simulink model "MMADC"  (R2021a)
settings: Solver=VariableStepAuto  StartTime=0.0  StopTime=1  RelTol=1e-3
values from neighbouring files (symbols this model uses):
  Cf = minimum_cap    [MMADC_main.m]
  clk_freq = 2.1*(nb_MAC+1)/nb_MAC*input_BW    (= 1684.375)    [MMADC_main.m]
  clk_period = 1/clk_freq    (= 0.000593692022263)    [MMADC_main.m]
  comparator_high_offset = 0.2*10e-4    (= 0.0002)    [MMADC_main.m]
  comparator_low_offset = -.1*10e-4    (= -0.0001)    [MMADC_main.m]
  comparator_noise_on = noise_on    (= 1)    [MMADC_main.m]
  comparator_noise_rms = 1*k*T* 2/3 / minimum_cap    [MMADC_main.m]
  comparator_offset_on = noise_on    (= 1)    [MMADC_main.m]
  k = 1.38064852e-23    [MMADC_main.m]
  LNA_bandwidth = 2.5*input_BW    (= 2000)    [MMADC_main.m]
  LNA_gain = 10^(36/20)*12*1.5849    (= 1200.00515432)    [MMADC_main.m]
  LNA_input_referred_noise = sqrt(pi/2*LNA_bandwidth*(194*10^-9)^2)    [MMADC_main.m]
  LNA_noise_on = noise_on    (= 1)    [MMADC_main.m]
  MM_incomplete_transfer_coeff = C1/(C1+C2)    [MMADC_main.m]
  MM_leakage_per_clk_cycle = 1    [MMADC_main.m]
  MM_sampling_noise = noise_on*((k*T * C1/(C1+C2)^2) + (k*T*(C1*C2/(C1+C2))/C2^2))    [MMADC_main.m]
  nb_MAC = 384    [MMADC_main.m]
  number_of_bits = 6    [MMADC_main.m]
  sample_time_jitter = 16e-12    (= 1.6e-11)    [MMADC_main.m]
  sampling_gain = Cs/Cf    [MMADC_main.m]
  sampling_jitter_on = noise_on    (= 1)    [MMADC_main.m]
  sensing_matrix = sensing_matrix_large(j:j+min(19,i-1),:)    [MMADC_main.m]
  sim_number = 0    [MMADC_main.m]
  switch_noise_on = noise_on    (= 1)    [MMADC_main.m]
  switching_noise = k*T/Cf    [MMADC_main.m]
  T = 293    [MMADC_main.m]
  Vref = 2    [MMADC_main.m]
  ZOH_delta = 0*Vref/(2^number_of_bits)    (= 0)    [MMADC_main.m]
libraries: simulink x100, simulink_extras x41, dspsigops x21, dspsrcs4 x21, spsFirstOrderFilterLib x1, dspswit3 x1
(part 9 of 10)

== system MMADC/Sensing Channel 2/SAR/ZOH+comparator/Old parallel ZOH comparator/Signal>DAC? ==
  y(t) : Inport
  DAC_in : Inport  Port=2
  Trigger : TriggerPort  VariantControl=Variant
  Add : Sum
  Add1 : Sum
  Compare To Zero : simulink/Logic and Bit Operations/Compare To Zero  relop=>  OutDataTypeStr=boolean
  Constant : Constant  Value=comparator_high_offset
  Constant1 : Constant  Value=comparator_low_offset
  Constant2 : Constant  Value=0
  Constant3 : Constant  Value=comparator_offset_on
  Constant4 : Constant  Value=0
  Constant5 : Constant  Value=comparator_noise_on
  Multiply : Gain  Gain=comparator_noise_rms
  Random Number : RandomNumber
  Subtract : Sum  Inputs=+-
  Switch : Switch  Criteria=u2 > Threshold
  Switch1 : Switch  Criteria=u2 > Threshold
  Switch2 : Switch  Criteria=u2 > Threshold
  Unit Delay : UnitDelay  SampleTime=-1  HasFrameUpgradeWarning=on
  Comparator_out : Outport
  wires:
  Switch/1 -> Switch1/1
  Subtract/1 -> Add/1
  Constant/1 -> Switch/1
  Constant2/1 -> Switch1/3
  Add/1 -> Compare To Zero/1
  Switch1/1 -> Add/2
  Compare To Zero/1 -> Unit Delay/1, Comparator_out/1
  Constant3/1 -> Switch1/2
  Unit Delay/1 -> Switch/2
  Constant1/1 -> Switch/3
  DAC_in/1 -> Subtract/2
  Add1/1 -> Subtract/1
  y(t)/1 -> Add1/2
  Random Number/1 -> Multiply/1
  Switch2/1 -> Add1/1
  Multiply/1 -> Switch2/1
  Constant4/1 -> Switch2/3
  Constant5/1 -> Switch2/2

== system MMADC/Sensing Channel 20/SAR/ZOH+comparator/Old parallel ZOH comparator/ DAC-signal < delta? ==
  y(t) : Inport
  DAC_in : Inport  Port=2
  Trigger : TriggerPort  VariantControl=Variant
  Add : Sum
  Add1 : Sum
  Compare To Zero : simulink/Logic and Bit Operations/Compare To Zero  relop=>  OutDataTypeStr=boolean
  Constant : Constant  Value=comparator_high_offset
  Constant1 : Constant  Value=comparator_low_offset
  Constant2 : Constant  Value=0
  Constant3 : Constant  Value=comparator_offset_on
  Constant4 : Constant  Value=0
  Constant5 : Constant  Value=comparator_noise_on
  Multiply : Gain  Gain=comparator_noise_rms
  Random Number : RandomNumber
  Subtract : Sum  Inputs=+-
  Switch : Switch  Criteria=u2 > Threshold
  Switch1 : Switch  Criteria=u2 > Threshold
  Switch2 : Switch  Criteria=u2 > Threshold
  Unit Delay : UnitDelay  SampleTime=-1  HasFrameUpgradeWarning=on
  Comparator_out : Outport
  wires:
  Switch/1 -> Switch1/1
  Subtract/1 -> Add/1
  Constant/1 -> Switch/1
  Constant2/1 -> Switch1/3
  Add/1 -> Compare To Zero/1
  Switch1/1 -> Add/2
  Compare To Zero/1 -> Unit Delay/1, Comparator_out/1
  Constant3/1 -> Switch1/2
  Unit Delay/1 -> Switch/2
  Constant1/1 -> Switch/3
  DAC_in/1 -> Subtract/2
  Add1/1 -> Subtract/1
  y(t)/1 -> Add1/2
  Random Number/1 -> Multiply/1
  Switch2/1 -> Add1/1
  Multiply/1 -> Switch2/1
  Constant4/1 -> Switch2/3
  Constant5/1 -> Switch2/2

== system MMADC/Sensing Channel 20/SAR/ZOH+comparator/Old parallel ZOH comparator/Count ZOH's ==
  In1 : Inport
  Trigger : TriggerPort  VariantControl=Variant  PortDimensions=1
  Add : Sum  AccumDataTypeStr=double  OutDataTypeStr=double
  Unit Delay : UnitDelay  SampleTime=-1  HasFrameUpgradeWarning=on
  Out1 : Outport
  wires:
  In1/1 -> Add/1
  Add/1 -> Unit Delay/1, Out1/1
  Unit Delay/1 -> Add/2

== system MMADC/Sensing Channel 20/SAR/ZOH+comparator/Old parallel ZOH comparator/Signal-DAC < delta? ==
  y(t) : Inport
  DAC_in : Inport  Port=2
  Trigger : TriggerPort  VariantControl=Variant
  Add : Sum
  Add1 : Sum
  Compare To Zero : simulink/Logic and Bit Operations/Compare To Zero  relop=>  OutDataTypeStr=boolean
  Constant : Constant  Value=comparator_high_offset
  Constant1 : Constant  Value=comparator_low_offset
  Constant2 : Constant  Value=0
  Constant3 : Constant  Value=comparator_offset_on
  Constant4 : Constant  Value=0
  Constant5 : Constant  Value=comparator_noise_on
  Multiply : Gain  Gain=comparator_noise_rms
  Random Number : RandomNumber
  Subtract : Sum  Inputs=+-
  Switch : Switch  Criteria=u2 > Threshold
  Switch1 : Switch  Criteria=u2 > Threshold
  Switch2 : Switch  Criteria=u2 > Threshold
  Unit Delay : UnitDelay  SampleTime=-1  HasFrameUpgradeWarning=on
  Comparator_out : Outport
  wires:
  Switch/1 -> Switch1/1
  Subtract/1 -> Add/1
  Constant/1 -> Switch/1
  Constant2/1 -> Switch1/3
  Add/1 -> Compare To Zero/1
  Switch1/1 -> Add/2
  Compare To Zero/1 -> Unit Delay/1, Comparator_out/1
  Constant3/1 -> Switch1/2
  Unit Delay/1 -> Switch/2
  Constant1/1 -> Switch/3
  DAC_in/1 -> Subtract/2
  Add1/1 -> Subtract/1
  y(t)/1 -> Add1/2
  Random Number/1 -> Multiply/1
  Switch2/1 -> Add1/1
  Multiply/1 -> Switch2/1
  Constant4/1 -> Switch2/3
  Constant5/1 -> Switch2/2

== system MMADC/Sensing Channel 20/SAR/ZOH+comparator/Old parallel ZOH comparator/Signal>DAC? ==
  y(t) : Inport
  DAC_in : Inport  Port=2
  Trigger : TriggerPort  VariantControl=Variant
  Add : Sum
  Add1 : Sum
  Compare To Zero : simulink/Logic and Bit Operations/Compare To Zero  relop=>  OutDataTypeStr=boolean
  Constant : Constant  Value=comparator_high_offset
  Constant1 : Constant  Value=comparator_low_offset
  Constant2 : Constant  Value=0
  Constant3 : Constant  Value=comparator_offset_on
  Constant4 : Constant  Value=0
  Constant5 : Constant  Value=comparator_noise_on
  Multiply : Gain  Gain=comparator_noise_rms
  Random Number : RandomNumber
  Subtract : Sum  Inputs=+-
  Switch : Switch  Criteria=u2 > Threshold
  Switch1 : Switch  Criteria=u2 > Threshold
  Switch2 : Switch  Criteria=u2 > Threshold
  Unit Delay : UnitDelay  SampleTime=-1  HasFrameUpgradeWarning=on
  Comparator_out : Outport
  wires:
  Switch/1 -> Switch1/1
  Subtract/1 -> Add/1
  Constant/1 -> Switch/1
  Constant2/1 -> Switch1/3
  Add/1 -> Compare To Zero/1
  Switch1/1 -> Add/2
  Compare To Zero/1 -> Unit Delay/1, Comparator_out/1
  Constant3/1 -> Switch1/2
  Unit Delay/1 -> Switch/2
  Constant1/1 -> Switch/3
  DAC_in/1 -> Subtract/2
  Add1/1 -> Subtract/1
  y(t)/1 -> Add1/2
  Random Number/1 -> Multiply/1
  Switch2/1 -> Add1/1
  Multiply/1 -> Switch2/1
  Constant4/1 -> Switch2/3
  Constant5/1 -> Switch2/2

== system MMADC/Sensing Channel 3/SAR/ZOH+comparator/Old parallel ZOH comparator/ DAC-signal < delta? ==
  y(t) : Inport
  DAC_in : Inport  Port=2
  Trigger : TriggerPort  VariantControl=Variant
  Add : Sum
  Add1 : Sum
  Compare To Zero : simulink/Logic and Bit Operations/Compare To Zero  relop=>  OutDataTypeStr=boolean
  Constant : Constant  Value=comparator_high_offset
  Constant1 : Constant  Value=comparator_low_offset
  Constant2 : Constant  Value=0
  Constant3 : Constant  Value=comparator_offset_on
  Constant4 : Constant  Value=0
  Constant5 : Constant  Value=comparator_noise_on
  Multiply : Gain  Gain=comparator_noise_rms
  Random Number : RandomNumber
  Subtract : Sum  Inputs=+-
  Switch : Switch  Criteria=u2 > Threshold
  Switch1 : Switch  Criteria=u2 > Threshold
  Switch2 : Switch  Criteria=u2 > Threshold
  Unit Delay : UnitDelay  SampleTime=-1  HasFrameUpgradeWarning=on
  Comparator_out : Outport
  wires:
  Switch/1 -> Switch1/1
  Subtract/1 -> Add/1
  Constant/1 -> Switch/1
  Constant2/1 -> Switch1/3
  Add/1 -> Compare To Zero/1
  Switch1/1 -> Add/2
  Compare To Zero/1 -> Unit Delay/1, Comparator_out/1
  Constant3/1 -> Switch1/2
  Unit Delay/1 -> Switch/2
  Constant1/1 -> Switch/3
  DAC_in/1 -> Subtract/2
  Add1/1 -> Subtract/1
  y(t)/1 -> Add1/2
  Random Number/1 -> Multiply/1
  Switch2/1 -> Add1/1
  Multiply/1 -> Switch2/1
  Constant4/1 -> Switch2/3
  Constant5/1 -> Switch2/2

== system MMADC/Sensing Channel 3/SAR/ZOH+comparator/Old parallel ZOH comparator/Count ZOH's ==
  In1 : Inport
  Trigger : TriggerPort  VariantControl=Variant  PortDimensions=1
  Add : Sum  AccumDataTypeStr=double  OutDataTypeStr=double
  Unit Delay : UnitDelay  SampleTime=-1  HasFrameUpgradeWarning=on
  Out1 : Outport
  wires:
  In1/1 -> Add/1
  Add/1 -> Unit Delay/1, Out1/1
  Unit Delay/1 -> Add/2

== system MMADC/Sensing Channel 3/SAR/ZOH+comparator/Old parallel ZOH comparator/Signal-DAC < delta? ==
  y(t) : Inport
  DAC_in : Inport  Port=2
  Trigger : TriggerPort  VariantControl=Variant
  Add : Sum
  Add1 : Sum
  Compare To Zero : simulink/Logic and Bit Operations/Compare To Zero  relop=>  OutDataTypeStr=boolean
  Constant : Constant  Value=comparator_high_offset
  Constant1 : Constant  Value=comparator_low_offset
  Constant2 : Constant  Value=0
  Constant3 : Constant  Value=comparator_offset_on
  Constant4 : Constant  Value=0
  Constant5 : Constant  Value=comparator_noise_on
  Multiply : Gain  Gain=comparator_noise_rms
  Random Number : RandomNumber
  Subtract : Sum  Inputs=+-
  Switch : Switch  Criteria=u2 > Threshold
  Switch1 : Switch  Criteria=u2 > Threshold
  Switch2 : Switch  Criteria=u2 > Threshold
  Unit Delay : UnitDelay  SampleTime=-1  HasFrameUpgradeWarning=on
  Comparator_out : Outport
  wires:
  Switch/1 -> Switch1/1
  Subtract/1 -> Add/1
  Constant/1 -> Switch/1
  Constant2/1 -> Switch1/3
  Add/1 -> Compare To Zero/1
  Switch1/1 -> Add/2
  Compare To Zero/1 -> Unit Delay/1, Comparator_out/1
  Constant3/1 -> Switch1/2
  Unit Delay/1 -> Switch/2
  Constant1/1 -> Switch/3
  DAC_in/1 -> Subtract/2
  Add1/1 -> Subtract/1
  y(t)/1 -> Add1/2
  Random Number/1 -> Multiply/1
  Switch2/1 -> Add1/1
  Multiply/1 -> Switch2/1
  Constant4/1 -> Switch2/3
  Constant5/1 -> Switch2/2

== system MMADC/Sensing Channel 3/SAR/ZOH+comparator/Old parallel ZOH comparator/Signal>DAC? ==
  y(t) : Inport
  DAC_in : Inport  Port=2
  Trigger : TriggerPort  VariantControl=Variant
  Add : Sum
  Add1 : Sum
  Compare To Zero : simulink/Logic and Bit Operations/Compare To Zero  relop=>  OutDataTypeStr=boolean
  Constant : Constant  Value=comparator_high_offset
  Constant1 : Constant  Value=comparator_low_offset
  Constant2 : Constant  Value=0
  Constant3 : Constant  Value=comparator_offset_on
  Constant4 : Constant  Value=0
  Constant5 : Constant  Value=comparator_noise_on
  Multiply : Gain  Gain=comparator_noise_rms
  Random Number : RandomNumber
  Subtract : Sum  Inputs=+-
  Switch : Switch  Criteria=u2 > Threshold
  Switch1 : Switch  Criteria=u2 > Threshold
  Switch2 : Switch  Criteria=u2 > Threshold
  Unit Delay : UnitDelay  SampleTime=-1  HasFrameUpgradeWarning=on
  Comparator_out : Outport
  wires:
  Switch/1 -> Switch1/1
  Subtract/1 -> Add/1
  Constant/1 -> Switch/1
  Constant2/1 -> Switch1/3
  Add/1 -> Compare To Zero/1
  Switch1/1 -> Add/2
  Compare To Zero/1 -> Unit Delay/1, Comparator_out/1
  Constant3/1 -> Switch1/2
  Unit Delay/1 -> Switch/2
  Constant1/1 -> Switch/3
  DAC_in/1 -> Subtract/2
  Add1/1 -> Subtract/1
  y(t)/1 -> Add1/2
  Random Number/1 -> Multiply/1
  Switch2/1 -> Add1/1
  Multiply/1 -> Switch2/1
  Constant4/1 -> Switch2/3
  Constant5/1 -> Switch2/2

== system MMADC/Sensing Channel 4/SAR/ZOH+comparator/Old parallel ZOH comparator/ DAC-signal < delta? ==
  y(t) : Inport
  DAC_in : Inport  Port=2
  Trigger : TriggerPort  VariantControl=Variant
  Add : Sum
  Add1 : Sum
  Compare To Zero : simulink/Logic and Bit Operations/Compare To Zero  relop=>  OutDataTypeStr=boolean
  Constant : Constant  Value=comparator_high_offset
  Constant1 : Constant  Value=comparator_low_offset
  Constant2 : Constant  Value=0
  Constant3 : Constant  Value=comparator_offset_on
  Constant4 : Constant  Value=0
  Constant5 : Constant  Value=comparator_noise_on
  Multiply : Gain  Gain=comparator_noise_rms
  Random Number : RandomNumber
  Subtract : Sum  Inputs=+-
  Switch : Switch  Criteria=u2 > Threshold
  Switch1 : Switch  Criteria=u2 > Threshold
  Switch2 : Switch  Criteria=u2 > Threshold
  Unit Delay : UnitDelay  SampleTime=-1  HasFrameUpgradeWarning=on
  Comparator_out : Outport
  wires:
  Switch/1 -> Switch1/1
  Subtract/1 -> Add/1
  Constant/1 -> Switch/1
  Constant2/1 -> Switch1/3
  Add/1 -> Compare To Zero/1
  Switch1/1 -> Add/2
  Compare To Zero/1 -> Unit Delay/1, Comparator_out/1
  Constant3/1 -> Switch1/2
  Unit Delay/1 -> Switch/2
  Constant1/1 -> Switch/3
  DAC_in/1 -> Subtract/2
  Add1/1 -> Subtract/1
  y(t)/1 -> Add1/2
  Random Number/1 -> Multiply/1
  Switch2/1 -> Add1/1
  Multiply/1 -> Switch2/1
  Constant4/1 -> Switch2/3
  Constant5/1 -> Switch2/2

== system MMADC/Sensing Channel 4/SAR/ZOH+comparator/Old parallel ZOH comparator/Count ZOH's ==
  In1 : Inport
  Trigger : TriggerPort  VariantControl=Variant  PortDimensions=1
  Add : Sum  AccumDataTypeStr=double  OutDataTypeStr=double
  Unit Delay : UnitDelay  SampleTime=-1  HasFrameUpgradeWarning=on
  Out1 : Outport
  wires:
  In1/1 -> Add/1
  Add/1 -> Unit Delay/1, Out1/1
  Unit Delay/1 -> Add/2

== system MMADC/Sensing Channel 4/SAR/ZOH+comparator/Old parallel ZOH comparator/Signal-DAC < delta? ==
  y(t) : Inport
  DAC_in : Inport  Port=2
  Trigger : TriggerPort  VariantControl=Variant
  Add : Sum
  Add1 : Sum
  Compare To Zero : simulink/Logic and Bit Operations/Compare To Zero  relop=>  OutDataTypeStr=boolean
  Constant : Constant  Value=comparator_high_offset
  Constant1 : Constant  Value=comparator_low_offset
  Constant2 : Constant  Value=0
  Constant3 : Constant  Value=comparator_offset_on
  Constant4 : Constant  Value=0
  Constant5 : Constant  Value=comparator_noise_on
  Multiply : Gain  Gain=comparator_noise_rms
  Random Number : RandomNumber
  Subtract : Sum  Inputs=+-
  Switch : Switch  Criteria=u2 > Threshold
  Switch1 : Switch  Criteria=u2 > Threshold
  Switch2 : Switch  Criteria=u2 > Threshold
  Unit Delay : UnitDelay  SampleTime=-1  HasFrameUpgradeWarning=on
  Comparator_out : Outport
  wires:
  Switch/1 -> Switch1/1
  Subtract/1 -> Add/1
  Constant/1 -> Switch/1
  Constant2/1 -> Switch1/3
  Add/1 -> Compare To Zero/1
  Switch1/1 -> Add/2
  Compare To Zero/1 -> Unit Delay/1, Comparator_out/1
  Constant3/1 -> Switch1/2
  Unit Delay/1 -> Switch/2
  Constant1/1 -> Switch/3
  DAC_in/1 -> Subtract/2
  Add1/1 -> Subtract/1
  y(t)/1 -> Add1/2
  Random Number/1 -> Multiply/1
  Switch2/1 -> Add1/1
  Multiply/1 -> Switch2/1
  Constant4/1 -> Switch2/3
  Constant5/1 -> Switch2/2

== system MMADC/Sensing Channel 4/SAR/ZOH+comparator/Old parallel ZOH comparator/Signal>DAC? ==
  y(t) : Inport
  DAC_in : Inport  Port=2
  Trigger : TriggerPort  VariantControl=Variant
  Add : Sum
  Add1 : Sum
  Compare To Zero : simulink/Logic and Bit Operations/Compare To Zero  relop=>  OutDataTypeStr=boolean
  Constant : Constant  Value=comparator_high_offset
  Constant1 : Constant  Value=comparator_low_offset
  Constant2 : Constant  Value=0
  Constant3 : Constant  Value=comparator_offset_on
  Constant4 : Constant  Value=0
  Constant5 : Constant  Value=comparator_noise_on
  Multiply : Gain  Gain=comparator_noise_rms
  Random Number : RandomNumber
  Subtract : Sum  Inputs=+-
  Switch : Switch  Criteria=u2 > Threshold
  Switch1 : Switch  Criteria=u2 > Threshold
  Switch2 : Switch  Criteria=u2 > Threshold
  Unit Delay : UnitDelay  SampleTime=-1  HasFrameUpgradeWarning=on
  Comparator_out : Outport
  wires:
  Switch/1 -> Switch1/1
  Subtract/1 -> Add/1
  Constant/1 -> Switch/1
  Constant2/1 -> Switch1/3
  Add/1 -> Compare To Zero/1
  Switch1/1 -> Add/2
  Compare To Zero/1 -> Unit Delay/1, Comparator_out/1
  Constant3/1 -> Switch1/2
  Unit Delay/1 -> Switch/2
  Constant1/1 -> Switch/3
  DAC_in/1 -> Subtract/2
  Add1/1 -> Subtract/1
  y(t)/1 -> Add1/2
  Random Number/1 -> Multiply/1
  Switch2/1 -> Add1/1
  Multiply/1 -> Switch2/1
  Constant4/1 -> Switch2/3
  Constant5/1 -> Switch2/2

== system MMADC/Sensing Channel 5/SAR/ZOH+comparator/Old parallel ZOH comparator/ DAC-signal < delta? ==
  y(t) : Inport
  DAC_in : Inport  Port=2
  Trigger : TriggerPort  VariantControl=Variant
  Add : Sum
  Add1 : Sum
  Compare To Zero : simulink/Logic and Bit Operations/Compare To Zero  relop=>  OutDataTypeStr=boolean
  Constant : Constant  Value=comparator_high_offset
  Constant1 : Constant  Value=comparator_low_offset
  Constant2 : Constant  Value=0
  Constant3 : Constant  Value=comparator_offset_on
  Constant4 : Constant  Value=0
  Constant5 : Constant  Value=comparator_noise_on
  Multiply : Gain  Gain=comparator_noise_rms
  Random Number : RandomNumber
  Subtract : Sum  Inputs=+-
  Switch : Switch  Criteria=u2 > Threshold
  Switch1 : Switch  Criteria=u2 > Threshold
  Switch2 : Switch  Criteria=u2 > Threshold
  Unit Delay : UnitDelay  SampleTime=-1  HasFrameUpgradeWarning=on
  Comparator_out : Outport
  wires:
  Switch/1 -> Switch1/1
  Subtract/1 -> Add/1
  Constant/1 -> Switch/1
  Constant2/1 -> Switch1/3
  Add/1 -> Compare To Zero/1
  Switch1/1 -> Add/2
  Compare To Zero/1 -> Unit Delay/1, Comparator_out/1
  Constant3/1 -> Switch1/2
  Unit Delay/1 -> Switch/2
  Constant1/1 -> Switch/3
  DAC_in/1 -> Subtract/2
  Add1/1 -> Subtract/1
  y(t)/1 -> Add1/2
  Random Number/1 -> Multiply/1
  Switch2/1 -> Add1/1
  Multiply/1 -> Switch2/1
  Constant4/1 -> Switch2/3
  Constant5/1 -> Switch2/2

== system MMADC/Sensing Channel 5/SAR/ZOH+comparator/Old parallel ZOH comparator/Count ZOH's ==
  In1 : Inport
  Trigger : TriggerPort  VariantControl=Variant  PortDimensions=1
  Add : Sum  AccumDataTypeStr=double  OutDataTypeStr=double
  Unit Delay : UnitDelay  SampleTime=-1  HasFrameUpgradeWarning=on
  Out1 : Outport
  wires:
  In1/1 -> Add/1
  Add/1 -> Unit Delay/1, Out1/1
  Unit Delay/1 -> Add/2

== system MMADC/Sensing Channel 5/SAR/ZOH+comparator/Old parallel ZOH comparator/Signal-DAC < delta? ==
  y(t) : Inport
  DAC_in : Inport  Port=2
  Trigger : TriggerPort  VariantControl=Variant
  Add : Sum
  Add1 : Sum
  Compare To Zero : simulink/Logic and Bit Operations/Compare To Zero  relop=>  OutDataTypeStr=boolean
  Constant : Constant  Value=comparator_high_offset
  Constant1 : Constant  Value=comparator_low_offset
  Constant2 : Constant  Value=0
  Constant3 : Constant  Value=comparator_offset_on
  Constant4 : Constant  Value=0
  Constant5 : Constant  Value=comparator_noise_on
  Multiply : Gain  Gain=comparator_noise_rms
  Random Number : RandomNumber
  Subtract : Sum  Inputs=+-
  Switch : Switch  Criteria=u2 > Threshold
  Switch1 : Switch  Criteria=u2 > Threshold
  Switch2 : Switch  Criteria=u2 > Threshold
  Unit Delay : UnitDelay  SampleTime=-1  HasFrameUpgradeWarning=on
  Comparator_out : Outport
  wires:
  Switch/1 -> Switch1/1
  Subtract/1 -> Add/1
  Constant/1 -> Switch/1
  Constant2/1 -> Switch1/3
  Add/1 -> Compare To Zero/1
  Switch1/1 -> Add/2
  Compare To Zero/1 -> Unit Delay/1, Comparator_out/1
  Constant3/1 -> Switch1/2
  Unit Delay/1 -> Switch/2
  Constant1/1 -> Switch/3
  DAC_in/1 -> Subtract/2
  Add1/1 -> Subtract/1
  y(t)/1 -> Add1/2
  Random Number/1 -> Multiply/1
  Switch2/1 -> Add1/1
  Multiply/1 -> Switch2/1
  Constant4/1 -> Switch2/3
  Constant5/1 -> Switch2/2

== system MMADC/Sensing Channel 5/SAR/ZOH+comparator/Old parallel ZOH comparator/Signal>DAC? ==
  y(t) : Inport
  DAC_in : Inport  Port=2
  Trigger : TriggerPort  VariantControl=Variant
  Add : Sum
  Add1 : Sum
  Compare To Zero : simulink/Logic and Bit Operations/Compare To Zero  relop=>  OutDataTypeStr=boolean
  Constant : Constant  Value=comparator_high_offset
  Constant1 : Constant  Value=comparator_low_offset
  Constant2 : Constant  Value=0
  Constant3 : Constant  Value=comparator_offset_on
  Constant4 : Constant  Value=0
  Constant5 : Constant  Value=comparator_noise_on
  Multiply : Gain  Gain=comparator_noise_rms
  Random Number : RandomNumber
  Subtract : Sum  Inputs=+-
  Switch : Switch  Criteria=u2 > Threshold
  Switch1 : Switch  Criteria=u2 > Threshold
  Switch2 : Switch  Criteria=u2 > Threshold
  Unit Delay : UnitDelay  SampleTime=-1  HasFrameUpgradeWarning=on
  Comparator_out : Outport
  wires:
  Switch/1 -> Switch1/1
  Subtract/1 -> Add/1
  Constant/1 -> Switch/1
  Constant2/1 -> Switch1/3
  Add/1 -> Compare To Zero/1
  Switch1/1 -> Add/2
  Compare To Zero/1 -> Unit Delay/1, Comparator_out/1
  Constant3/1 -> Switch1/2
  Unit Delay/1 -> Switch/2
  Constant1/1 -> Switch/3
  DAC_in/1 -> Subtract/2
  Add1/1 -> Subtract/1
  y(t)/1 -> Add1/2
  Random Number/1 -> Multiply/1
  Switch2/1 -> Add1/1
  Multiply/1 -> Switch2/1
  Constant4/1 -> Switch2/3
  Constant5/1 -> Switch2/2

== system MMADC/Sensing Channel 6/SAR/ZOH+comparator/Old parallel ZOH comparator/ DAC-signal < delta? ==
  y(t) : Inport
  DAC_in : Inport  Port=2
  Trigger : TriggerPort  VariantControl=Variant
  Add : Sum
  Add1 : Sum
  Compare To Zero : simulink/Logic and Bit Operations/Compare To Zero  relop=>  OutDataTypeStr=boolean
  Constant : Constant  Value=comparator_high_offset
  Constant1 : Constant  Value=comparator_low_offset
  Constant2 : Constant  Value=0
  Constant3 : Constant  Value=comparator_offset_on
  Constant4 : Constant  Value=0
  Constant5 : Constant  Value=comparator_noise_on
  Multiply : Gain  Gain=comparator_noise_rms
  Random Number : RandomNumber
  Subtract : Sum  Inputs=+-
  Switch : Switch  Criteria=u2 > Threshold
  Switch1 : Switch  Criteria=u2 > Threshold
  Switch2 : Switch  Criteria=u2 > Threshold
  Unit Delay : UnitDelay  SampleTime=-1  HasFrameUpgradeWarning=on
  Comparator_out : Outport
  wires:
  Switch/1 -> Switch1/1
  Subtract/1 -> Add/1
  Constant/1 -> Switch/1
  Constant2/1 -> Switch1/3
  Add/1 -> Compare To Zero/1
  Switch1/1 -> Add/2
  Compare To Zero/1 -> Unit Delay/1, Comparator_out/1
  Constant3/1 -> Switch1/2
  Unit Delay/1 -> Switch/2
  Constant1/1 -> Switch/3
  DAC_in/1 -> Subtract/2
  Add1/1 -> Subtract/1
  y(t)/1 -> Add1/2
  Random Number/1 -> Multiply/1
  Switch2/1 -> Add1/1
  Multiply/1 -> Switch2/1
  Constant4/1 -> Switch2/3
  Constant5/1 -> Switch2/2

== system MMADC/Sensing Channel 6/SAR/ZOH+comparator/Old parallel ZOH comparator/Count ZOH's ==
  In1 : Inport
  Trigger : TriggerPort  VariantControl=Variant  PortDimensions=1
  Add : Sum  AccumDataTypeStr=double  OutDataTypeStr=double
  Unit Delay : UnitDelay  SampleTime=-1  HasFrameUpgradeWarning=on
  Out1 : Outport
  wires:
  In1/1 -> Add/1
  Add/1 -> Unit Delay/1, Out1/1
  Unit Delay/1 -> Add/2

== system MMADC/Sensing Channel 6/SAR/ZOH+comparator/Old parallel ZOH comparator/Signal-DAC < delta? ==
  y(t) : Inport
  DAC_in : Inport  Port=2
  Trigger : TriggerPort  VariantControl=Variant
  Add : Sum
  Add1 : Sum
  Compare To Zero : simulink/Logic and Bit Operations/Compare To Zero  relop=>  OutDataTypeStr=boolean
  Constant : Constant  Value=comparator_high_offset
  Constant1 : Constant  Value=comparator_low_offset
  Constant2 : Constant  Value=0
  Constant3 : Constant  Value=comparator_offset_on
  Constant4 : Constant  Value=0
  Constant5 : Constant  Value=comparator_noise_on
  Multiply : Gain  Gain=comparator_noise_rms
  Random Number : RandomNumber
  Subtract : Sum  Inputs=+-
  Switch : Switch  Criteria=u2 > Threshold
  Switch1 : Switch  Criteria=u2 > Threshold
  Switch2 : Switch  Criteria=u2 > Threshold
  Unit Delay : UnitDelay  SampleTime=-1  HasFrameUpgradeWarning=on
  Comparator_out : Outport
  wires:
  Switch/1 -> Switch1/1
  Subtract/1 -> Add/1
  Constant/1 -> Switch/1
  Constant2/1 -> Switch1/3
  Add/1 -> Compare To Zero/1
  Switch1/1 -> Add/2
  Compare To Zero/1 -> Unit Delay/1, Comparator_out/1
  Constant3/1 -> Switch1/2
  Unit Delay/1 -> Switch/2
  Constant1/1 -> Switch/3
  DAC_in/1 -> Subtract/2
  Add1/1 -> Subtract/1
  y(t)/1 -> Add1/2
  Random Number/1 -> Multiply/1
  Switch2/1 -> Add1/1
  Multiply/1 -> Switch2/1
  Constant4/1 -> Switch2/3
  Constant5/1 -> Switch2/2

== system MMADC/Sensing Channel 6/SAR/ZOH+comparator/Old parallel ZOH comparator/Signal>DAC? ==
  y(t) : Inport
  DAC_in : Inport  Port=2
  Trigger : TriggerPort  VariantControl=Variant
  Add : Sum
  Add1 : Sum
  Compare To Zero : simulink/Logic and Bit Operations/Compare To Zero  relop=>  OutDataTypeStr=boolean
  Constant : Constant  Value=comparator_high_offset
  Constant1 : Constant  Value=comparator_low_offset
  Constant2 : Constant  Value=0
  Constant3 : Constant  Value=comparator_offset_on
  Constant4 : Constant  Value=0
  Constant5 : Constant  Value=comparator_noise_on
  Multiply : Gain  Gain=comparator_noise_rms
  Random Number : RandomNumber
  Subtract : Sum  Inputs=+-
  Switch : Switch  Criteria=u2 > Threshold
  Switch1 : Switch  Criteria=u2 > Threshold
  Switch2 : Switch  Criteria=u2 > Threshold
  Unit Delay : UnitDelay  SampleTime=-1  HasFrameUpgradeWarning=on
  Comparator_out : Outport
  wires:
  Switch/1 -> Switch1/1
  Subtract/1 -> Add/1
  Constant/1 -> Switch/1
  Constant2/1 -> Switch1/3
  Add/1 -> Compare To Zero/1
  Switch1/1 -> Add/2
  Compare To Zero/1 -> Unit Delay/1, Comparator_out/1
  Constant3/1 -> Switch1/2
  Unit Delay/1 -> Switch/2
  Constant1/1 -> Switch/3
  DAC_in/1 -> Subtract/2
  Add1/1 -> Subtract/1
  y(t)/1 -> Add1/2
  Random Number/1 -> Multiply/1
  Switch2/1 -> Add1/1
  Multiply/1 -> Switch2/1
  Constant4/1 -> Switch2/3
  Constant5/1 -> Switch2/2

== system MMADC/Sensing Channel 7/SAR/ZOH+comparator/Old parallel ZOH comparator/ DAC-signal < delta? ==
  y(t) : Inport
  DAC_in : Inport  Port=2
  Trigger : TriggerPort  VariantControl=Variant
  Add : Sum
  Add1 : Sum
  Compare To Zero : simulink/Logic and Bit Operations/Compare To Zero  relop=>  OutDataTypeStr=boolean
  Constant : Constant  Value=comparator_high_offset
  Constant1 : Constant  Value=comparator_low_offset
  Constant2 : Constant  Value=0
  Constant3 : Constant  Value=comparator_offset_on
  Constant4 : Constant  Value=0
  Constant5 : Constant  Value=comparator_noise_on
  Multiply : Gain  Gain=comparator_noise_rms
  Random Number : RandomNumber
  Subtract : Sum  Inputs=+-
  Switch : Switch  Criteria=u2 > Threshold
  Switch1 : Switch  Criteria=u2 > Threshold
  Switch2 : Switch  Criteria=u2 > Threshold
  Unit Delay : UnitDelay  SampleTime=-1  HasFrameUpgradeWarning=on
  Comparator_out : Outport
  wires:
  Switch/1 -> Switch1/1
  Subtract/1 -> Add/1
  Constant/1 -> Switch/1
  Constant2/1 -> Switch1/3
  Add/1 -> Compare To Zero/1
  Switch1/1 -> Add/2
  Compare To Zero/1 -> Unit Delay/1, Comparator_out/1
  Constant3/1 -> Switch1/2
  Unit Delay/1 -> Switch/2
  Constant1/1 -> Switch/3
  DAC_in/1 -> Subtract/2
  Add1/1 -> Subtract/1
  y(t)/1 -> Add1/2
  Random Number/1 -> Multiply/1
  Switch2/1 -> Add1/1
  Multiply/1 -> Switch2/1
  Constant4/1 -> Switch2/3
  Constant5/1 -> Switch2/2

== system MMADC/Sensing Channel 7/SAR/ZOH+comparator/Old parallel ZOH comparator/Count ZOH's ==
  In1 : Inport
  Trigger : TriggerPort  VariantControl=Variant  PortDimensions=1
  Add : Sum  AccumDataTypeStr=double  OutDataTypeStr=double
  Unit Delay : UnitDelay  SampleTime=-1  HasFrameUpgradeWarning=on
  Out1 : Outport
  wires:
  In1/1 -> Add/1
  Add/1 -> Unit Delay/1, Out1/1
  Unit Delay/1 -> Add/2

== system MMADC/Sensing Channel 7/SAR/ZOH+comparator/Old parallel ZOH comparator/Signal-DAC < delta? ==
  y(t) : Inport
  DAC_in : Inport  Port=2
  Trigger : TriggerPort  VariantControl=Variant
  Add : Sum
  Add1 : Sum
  Compare To Zero : simulink/Logic and Bit Operations/Compare To Zero  relop=>  OutDataTypeStr=boolean
  Constant : Constant  Value=comparator_high_offset
  Constant1 : Constant  Value=comparator_low_offset
  Constant2 : Constant  Value=0
  Constant3 : Constant  Value=comparator_offset_on
  Constant4 : Constant  Value=0
  Constant5 : Constant  Value=comparator_noise_on
  Multiply : Gain  Gain=comparator_noise_rms
  Random Number : RandomNumber
  Subtract : Sum  Inputs=+-
  Switch : Switch  Criteria=u2 > Threshold
  Switch1 : Switch  Criteria=u2 > Threshold
  Switch2 : Switch  Criteria=u2 > Threshold
  Unit Delay : UnitDelay  SampleTime=-1  HasFrameUpgradeWarning=on
  Comparator_out : Outport
  wires:
  Switch/1 -> Switch1/1
  Subtract/1 -> Add/1
  Constant/1 -> Switch/1
  Constant2/1 -> Switch1/3
  Add/1 -> Compare To Zero/1
  Switch1/1 -> Add/2
  Compare To Zero/1 -> Unit Delay/1, Comparator_out/1
  Constant3/1 -> Switch1/2
  Unit Delay/1 -> Switch/2
  Constant1/1 -> Switch/3
  DAC_in/1 -> Subtract/2
  Add1/1 -> Subtract/1
  y(t)/1 -> Add1/2
  Random Number/1 -> Multiply/1
  Switch2/1 -> Add1/1
  Multiply/1 -> Switch2/1
  Constant4/1 -> Switch2/3
  Constant5/1 -> Switch2/2

== system MMADC/Sensing Channel 7/SAR/ZOH+comparator/Old parallel ZOH comparator/Signal>DAC? ==
  y(t) : Inport
  DAC_in : Inport  Port=2
  Trigger : TriggerPort  VariantControl=Variant
  Add : Sum
  Add1 : Sum
  Compare To Zero : simulink/Logic and Bit Operations/Compare To Zero  relop=>  OutDataTypeStr=boolean
  Constant : Constant  Value=comparator_high_offset
  Constant1 : Constant  Value=comparator_low_offset
  Constant2 : Constant  Value=0
  Constant3 : Constant  Value=comparator_offset_on
  Constant4 : Constant  Value=0
  Constant5 : Constant  Value=comparator_noise_on
  Multiply : Gain  Gain=comparator_noise_rms
  Random Number : RandomNumber
  Subtract : Sum  Inputs=+-
  Switch : Switch  Criteria=u2 > Threshold
  Switch1 : Switch  Criteria=u2 > Threshold
  Switch2 : Switch  Criteria=u2 > Threshold
  Unit Delay : UnitDelay  SampleTime=-1  HasFrameUpgradeWarning=on
  Comparator_out : Outport
  wires:
  Switch/1 -> Switch1/1
  Subtract/1 -> Add/1
  Constant/1 -> Switch/1
  Constant2/1 -> Switch1/3
  Add/1 -> Compare To Zero/1
  Switch1/1 -> Add/2
  Compare To Zero/1 -> Unit Delay/1, Comparator_out/1
  Constant3/1 -> Switch1/2
  Unit Delay/1 -> Switch/2
  Constant1/1 -> Switch/3
  DAC_in/1 -> Subtract/2
  Add1/1 -> Subtract/1
  y(t)/1 -> Add1/2
  Random Number/1 -> Multiply/1
  Switch2/1 -> Add1/1
  Multiply/1 -> Switch2/1
  Constant4/1 -> Switch2/3
  Constant5/1 -> Switch2/2

== system MMADC/Sensing Channel 8/SAR/ZOH+comparator/Old parallel ZOH comparator/ DAC-signal < delta? ==
  y(t) : Inport
  DAC_in : Inport  Port=2
  Trigger : TriggerPort  VariantControl=Variant
  Add : Sum
  Add1 : Sum
  Compare To Zero : simulink/Logic and Bit Operations/Compare To Zero  relop=>  OutDataTypeStr=boolean
  Constant : Constant  Value=comparator_high_offset
  Constant1 : Constant  Value=comparator_low_offset
  Constant2 : Constant  Value=0
  Constant3 : Constant  Value=comparator_offset_on
  Constant4 : Constant  Value=0
  Constant5 : Constant  Value=comparator_noise_on
  Multiply : Gain  Gain=comparator_noise_rms
  Random Number : RandomNumber
  Subtract : Sum  Inputs=+-
  Switch : Switch  Criteria=u2 > Threshold
  Switch1 : Switch  Criteria=u2 > Threshold
  Switch2 : Switch  Criteria=u2 > Threshold
  Unit Delay : UnitDelay  SampleTime=-1  HasFrameUpgradeWarning=on
  Comparator_out : Outport
  wires:
  Switch/1 -> Switch1/1
  Subtract/1 -> Add/1
  Constant/1 -> Switch/1
  Constant2/1 -> Switch1/3
  Add/1 -> Compare To Zero/1
  Switch1/1 -> Add/2
  Compare To Zero/1 -> Unit Delay/1, Comparator_out/1
  Constant3/1 -> Switch1/2
  Unit Delay/1 -> Switch/2
  Constant1/1 -> Switch/3
  DAC_in/1 -> Subtract/2
  Add1/1 -> Subtract/1
  y(t)/1 -> Add1/2
  Random Number/1 -> Multiply/1
  Switch2/1 -> Add1/1
  Multiply/1 -> Switch2/1
  Constant4/1 -> Switch2/3
  Constant5/1 -> Switch2/2

== system MMADC/Sensing Channel 8/SAR/ZOH+comparator/Old parallel ZOH comparator/Count ZOH's ==
  In1 : Inport
  Trigger : TriggerPort  VariantControl=Variant  PortDimensions=1
  Add : Sum  AccumDataTypeStr=double  OutDataTypeStr=double
  Unit Delay : UnitDelay  SampleTime=-1  HasFrameUpgradeWarning=on
  Out1 : Outport
  wires:
  In1/1 -> Add/1
  Add/1 -> Unit Delay/1, Out1/1
  Unit Delay/1 -> Add/2

== system MMADC/Sensing Channel 8/SAR/ZOH+comparator/Old parallel ZOH comparator/Signal-DAC < delta? ==
  y(t) : Inport
  DAC_in : Inport  Port=2
  Trigger : TriggerPort  VariantControl=Variant
  Add : Sum
  Add1 : Sum
  Compare To Zero : simulink/Logic and Bit Operations/Compare To Zero  relop=>  OutDataTypeStr=boolean
  Constant : Constant  Value=comparator_high_offset
  Constant1 : Constant  Value=comparator_low_offset
  Constant2 : Constant  Value=0
  Constant3 : Constant  Value=comparator_offset_on
  Constant4 : Constant  Value=0
  Constant5 : Constant  Value=comparator_noise_on
  Multiply : Gain  Gain=comparator_noise_rms
  Random Number : RandomNumber
  Subtract : Sum  Inputs=+-
  Switch : Switch  Criteria=u2 > Threshold
  Switch1 : Switch  Criteria=u2 > Threshold
  Switch2 : Switch  Criteria=u2 > Threshold
  Unit Delay : UnitDelay  SampleTime=-1  HasFrameUpgradeWarning=on
  Comparator_out : Outport
  wires:
  Switch/1 -> Switch1/1
  Subtract/1 -> Add/1
  Constant/1 -> Switch/1
  Constant2/1 -> Switch1/3
  Add/1 -> Compare To Zero/1
  Switch1/1 -> Add/2
  Compare To Zero/1 -> Unit Delay/1, Comparator_out/1
  Constant3/1 -> Switch1/2
  Unit Delay/1 -> Switch/2
  Constant1/1 -> Switch/3
  DAC_in/1 -> Subtract/2
  Add1/1 -> Subtract/1
  y(t)/1 -> Add1/2
  Random Number/1 -> Multiply/1
  Switch2/1 -> Add1/1
  Multiply/1 -> Switch2/1
  Constant4/1 -> Switch2/3
  Constant5/1 -> Switch2/2

== system MMADC/Sensing Channel 8/SAR/ZOH+comparator/Old parallel ZOH comparator/Signal>DAC? ==
  y(t) : Inport
  DAC_in : Inport  Port=2
  Trigger : TriggerPort  VariantControl=Variant
  Add : Sum
  Add1 : Sum
  Compare To Zero : simulink/Logic and Bit Operations/Compare To Zero  relop=>  OutDataTypeStr=boolean
  Constant : Constant  Value=comparator_high_offset
  Constant1 : Constant  Value=comparator_low_offset
  Constant2 : Constant  Value=0
  Constant3 : Constant  Value=comparator_offset_on
  Constant4 : Constant  Value=0
  Constant5 : Constant  Value=comparator_noise_on
  Multiply : Gain  Gain=comparator_noise_rms
  Random Number : RandomNumber
  Subtract : Sum  Inputs=+-
  Switch : Switch  Criteria=u2 > Threshold
  Switch1 : Switch  Criteria=u2 > Threshold
  Switch2 : Switch  Criteria=u2 > Threshold
  Unit Delay : UnitDelay  SampleTime=-1  HasFrameUpgradeWarning=on
  Comparator_out : Outport
  wires:
  Switch/1 -> Switch1/1
  Subtract/1 -> Add/1
  Constant/1 -> Switch/1
  Constant2/1 -> Switch1/3
  Add/1 -> Compare To Zero/1
  Switch1/1 -> Add/2
  Compare To Zero/1 -> Unit Delay/1, Comparator_out/1
  Constant3/1 -> Switch1/2
  Unit Delay/1 -> Switch/2
  Constant1/1 -> Switch/3
  DAC_in/1 -> Subtract/2
  Add1/1 -> Subtract/1
  y(t)/1 -> Add1/2
  Random Number/1 -> Multiply/1
  Switch2/1 -> Add1/1
  Multiply/1 -> Switch2/1
  Constant4/1 -> Switch2/3
  Constant5/1 -> Switch2/2

== system MMADC/Sensing Channel 9/SAR/ZOH+comparator/Old parallel ZOH comparator/ DAC-signal < delta? ==
  y(t) : Inport
  DAC_in : Inport  Port=2
  Trigger : TriggerPort  VariantControl=Variant
  Add : Sum
  Add1 : Sum
  Compare To Zero : simulink/Logic and Bit Operations/Compare To Zero  relop=>  OutDataTypeStr=boolean
  Constant : Constant  Value=comparator_high_offset
  Constant1 : Constant  Value=comparator_low_offset
  Constant2 : Constant  Value=0
  Constant3 : Constant  Value=comparator_offset_on
  Constant4 : Constant  Value=0
  Constant5 : Constant  Value=comparator_noise_on
  Multiply : Gain  Gain=comparator_noise_rms
  Random Number : RandomNumber
  Subtract : Sum  Inputs=+-
  Switch : Switch  Criteria=u2 > Threshold
  Switch1 : Switch  Criteria=u2 > Threshold
  Switch2 : Switch  Criteria=u2 > Threshold
  Unit Delay : UnitDelay  SampleTime=-1  HasFrameUpgradeWarning=on
  Comparator_out : Outport
  wires:
  Switch/1 -> Switch1/1
  Subtract/1 -> Add/1
  Constant/1 -> Switch/1
  Constant2/1 -> Switch1/3
  Add/1 -> Compare To Zero/1
  Switch1/1 -> Add/2
  Compare To Zero/1 -> Unit Delay/1, Comparator_out/1
  Constant3/1 -> Switch1/2
  Unit Delay/1 -> Switch/2
  Constant1/1 -> Switch/3
  DAC_in/1 -> Subtract/2
  Add1/1 -> Subtract/1
  y(t)/1 -> Add1/2
  Random Number/1 -> Multiply/1
  Switch2/1 -> Add1/1
  Multiply/1 -> Switch2/1
  Constant4/1 -> Switch2/3
  Constant5/1 -> Switch2/2

== system MMADC/Sensing Channel 9/SAR/ZOH+comparator/Old parallel ZOH comparator/Count ZOH's ==
  In1 : Inport
  Trigger : TriggerPort  VariantControl=Variant  PortDimensions=1
  Add : Sum  AccumDataTypeStr=double  OutDataTypeStr=double
  Unit Delay : UnitDelay  SampleTime=-1  HasFrameUpgradeWarning=on
  Out1 : Outport
  wires:
  In1/1 -> Add/1
  Add/1 -> Unit Delay/1, Out1/1
  Unit Delay/1 -> Add/2

== system MMADC/Sensing Channel 9/SAR/ZOH+comparator/Old parallel ZOH comparator/Signal-DAC < delta? ==
  y(t) : Inport
  DAC_in : Inport  Port=2
  Trigger : TriggerPort  VariantControl=Variant
  Add : Sum
  Add1 : Sum
  Compare To Zero : simulink/Logic and Bit Operations/Compare To Zero  relop=>  OutDataTypeStr=boolean
  Constant : Constant  Value=comparator_high_offset
  Constant1 : Constant  Value=comparator_low_offset
  Constant2 : Constant  Value=0
  Constant3 : Constant  Value=comparator_offset_on
  Constant4 : Constant  Value=0
  Constant5 : Constant  Value=comparator_noise_on
  Multiply : Gain  Gain=comparator_noise_rms
  Random Number : RandomNumber
  Subtract : Sum  Inputs=+-
  Switch : Switch  Criteria=u2 > Threshold
  Switch1 : Switch  Criteria=u2 > Threshold
  Switch2 : Switch  Criteria=u2 > Threshold
  Unit Delay : UnitDelay  SampleTime=-1  HasFrameUpgradeWarning=on
  Comparator_out : Outport
  wires:
  Switch/1 -> Switch1/1
  Subtract/1 -> Add/1
  Constant/1 -> Switch/1
  Constant2/1 -> Switch1/3
  Add/1 -> Compare To Zero/1
  Switch1/1 -> Add/2
  Compare To Zero/1 -> Unit Delay/1, Comparator_out/1
  Constant3/1 -> Switch1/2
  Unit Delay/1 -> Switch/2
  Constant1/1 -> Switch/3
  DAC_in/1 -> Subtract/2
  Add1/1 -> Subtract/1
  y(t)/1 -> Add1/2
  Random Number/1 -> Multiply/1
  Switch2/1 -> Add1/1
  Multiply/1 -> Switch2/1
  Constant4/1 -> Switch2/3
  Constant5/1 -> Switch2/2

== system MMADC/Sensing Channel 9/SAR/ZOH+comparator/Old parallel ZOH comparator/Signal>DAC? ==
  y(t) : Inport
  DAC_in : Inport  Port=2
  Trigger : TriggerPort  VariantControl=Variant
  Add : Sum
  Add1 : Sum
  Compare To Zero : simulink/Logic and Bit Operations/Compare To Zero  relop=>  OutDataTypeStr=boolean
  Constant : Constant  Value=comparator_high_offset
  Constant1 : Constant  Value=comparator_low_offset
  Constant2 : Constant  Value=0
  Constant3 : Constant  Value=comparator_offset_on
  Constant4 : Constant  Value=0
  Constant5 : Constant  Value=comparator_noise_on
  Multiply : Gain  Gain=comparator_noise_rms
  Random Number : RandomNumber
  Subtract : Sum  Inputs=+-
  Switch : Switch  Criteria=u2 > Threshold
  Switch1 : Switch  Criteria=u2 > Threshold
  Switch2 : Switch  Criteria=u2 > Threshold
  Unit Delay : UnitDelay  SampleTime=-1  HasFrameUpgradeWarning=on
  Comparator_out : Outport
  wires:
  Switch/1 -> Switch1/1
  Subtract/1 -> Add/1
  Constant/1 -> Switch/1
  Constant2/1 -> Switch1/3
  Add/1 -> Compare To Zero/1
  Switch1/1 -> Add/2
  Compare To Zero/1 -> Unit Delay/1, Comparator_out/1
  Constant3/1 -> Switch1/2
  Unit Delay/1 -> Switch/2
  Constant1/1 -> Switch/3
  DAC_in/1 -> Subtract/2
  Add1/1 -> Subtract/1
  y(t)/1 -> Add1/2
  Random Number/1 -> Multiply/1
  Switch2/1 -> Add1/1
  Multiply/1 -> Switch2/1
  Constant4/1 -> Switch2/3
  Constant5/1 -> Switch2/2

== matlab function MMADC/Sensing Channel 3/SAR/SAR/SAR ==
  data: output_code_decimal output size=1; cycle_out output size=1; output_code output size=number_of_bits; input_code_decimal input; cycle_in input; comparator_in input; number_of_bits input; done output; ZOH_true input
function [output_code_decimal, cycle_out, output_code, done] = fcn(input_code_decimal, cycle_in, comparator_in, number_of_bits, ZOH_true)

    input_code = de2bi(input_code_decimal, 'left-msb');
    output_code = [zeros(number_of_bits-size(input_code.',1),1); input_code.'];
    cycle_out = cycle_in + 1;
    done = 0;

    if (cycle_in < 2)
        
        % Wait for ZOH to be determined
        
    elseif (cycle_in == 2)
        % Reset output code, start SA algorithm unless ZOH
        if (~ZOH_true)
            output_code = zeros(number_of_bits,1);
            output_code(1, 1) = 1;
        end
        
    elseif (cycle_in == number_of_bits+2)
        % Finish SA algorithm unless ZOH, set done & reset output_cycle
        done = 1;
        if (~ZOH_true)
            output_code(number_of_bits,1) = comparator_in;
        end
        cycle_out = 0;
    else
        % Continue SA algorithm unless ZOH
        if (~ZOH_true)
            if (comparator_in == 0)
                output_code(cycle_in-2,1) = 0;
            end

            output_code(cycle_in-1,1) = 1;
        end
        
    end
    
    output_code_decimal_temp = bi2de(output_code.', 'left-msb');
    output_code_decimal = output_code_decimal_temp(1,1);
end

== matlab function MMADC/Sensing Channel 3/SAR/ZOH+comparator/MATLAB Function ==
  data: SAR_clk_cycle input; y output
function y = fcn(SAR_clk_cycle)
    if (SAR_clk_cycle)==0
        y = 2;
    elseif (SAR_clk_cycle)==1
        y=3;
    else
        y=1;
    end
end

== matlab function MMADC/Sensing Channel 4/SAR/DAC/DAC ==
  data: input_code input size=number_of_bits; out output double size=1; number_of_bits input; Vref input
function out = fcn(input_code, number_of_bits, Vref)
out = -Vref/2 + Vref/(2^number_of_bits) * (bi2de(input_code.', 'left-msb'));
end

== matlab function MMADC/Sensing Channel 4/SAR/SAR/SAR ==
  data: output_code_decimal output size=1; cycle_out output size=1; output_code output size=number_of_bits; input_code_decimal input; cycle_in input; comparator_in input; number_of_bits input; done output; ZOH_true input
function [output_code_decimal, cycle_out, output_code, done] = fcn(input_code_decimal, cycle_in, comparator_in, number_of_bits, ZOH_true)

    input_code = de2bi(input_code_decimal, 'left-msb');
    output_code = [zeros(number_of_bits-size(input_code.',1),1); input_code.'];
    cycle_out = cycle_in + 1;
    done = 0;

    if (cycle_in < 2)
        
        % Wait for ZOH to be determined
        
    elseif (cycle_in == 2)
        % Reset output code, start SA algorithm unless ZOH
        if (~ZOH_true)
            output_code = zeros(number_of_bits,1);
            output_code(1, 1) = 1;
        end
        
    elseif (cycle_in == number_of_bits+2)
        % Finish SA algorithm unless ZOH, set done & reset output_cycle
        done = 1;
        if (~ZOH_true)
            output_code(number_of_bits,1) = comparator_in;
        end
        cycle_out = 0;
    else
        % Continue SA algorithm unless ZOH
        if (~ZOH_true)
            if (comparator_in == 0)
                output_code(cycle_in-2,1) = 0;
            end

            output_code(cycle_in-1,1) = 1;
        end
        
    end
    
    output_code_decimal_temp = bi2de(output_code.', 'left-msb');
    output_code_decimal = output_code_decimal_temp(1,1);
end

== matlab function MMADC/Sensing Channel 4/SAR/ZOH+comparator/MATLAB Function ==
  data: SAR_clk_cycle input; y output
function y = fcn(SAR_clk_cycle)
    if (SAR_clk_cycle)==0
        y = 2;
    elseif (SAR_clk_cycle)==1
        y=3;
    else
        y=1;
    end
end

== matlab function MMADC/Sensing Channel 5/SAR/DAC/DAC ==
  data: input_code input size=number_of_bits; out output double size=1; number_of_bits input; Vref input
function out = fcn(input_code, number_of_bits, Vref)
out = -Vref/2 + Vref/(2^number_of_bits) * (bi2de(input_code.', 'left-msb'));
end

== matlab function MMADC/Sensing Channel 5/SAR/SAR/SAR ==
  data: output_code_decimal output size=1; cycle_out output size=1; output_code output size=number_of_bits; input_code_decimal input; cycle_in input; comparator_in input; number_of_bits input; done output; ZOH_true input
function [output_code_decimal, cycle_out, output_code, done] = fcn(input_code_decimal, cycle_in, comparator_in, number_of_bits, ZOH_true)

    input_code = de2bi(input_code_decimal, 'left-msb');
    output_code = [zeros(number_of_bits-size(input_code.',1),1); input_code.'];
    cycle_out = cycle_in + 1;
    done = 0;

    if (cycle_in < 2)
        
        % Wait for ZOH to be determined
        
    elseif (cycle_in == 2)
        % Reset output code, start SA algorithm unless ZOH
        if (~ZOH_true)
            output_code = zeros(number_of_bits,1);
            output_code(1, 1) = 1;
        end
        
    elseif (cycle_in == number_of_bits+2)
        % Finish SA algorithm unless ZOH, set done & reset output_cycle
        done = 1;
        if (~ZOH_true)
            output_code(number_of_bits,1) = comparator_in;
        end
        cycle_out = 0;
    else
        % Continue SA algorithm unless ZOH
        if (~ZOH_true)
            if (comparator_in == 0)
                output_code(cycle_in-2,1) = 0;
            end

            output_code(cycle_in-1,1) = 1;
        end
        
    end
    
    output_code_decimal_temp = bi2de(output_code.', 'left-msb');
    output_code_decimal = output_code_decimal_temp(1,1);
end

== matlab function MMADC/Sensing Channel 5/SAR/ZOH+comparator/MATLAB Function ==
  data: SAR_clk_cycle input; y output
function y = fcn(SAR_clk_cycle)
    if (SAR_clk_cycle)==0
        y = 2;
    elseif (SAR_clk_cycle)==1
        y=3;
    else
        y=1;
    end
end

== matlab function MMADC/Sensing Channel 6/SAR/DAC/DAC ==
  data: input_code input size=number_of_bits; out output double size=1; number_of_bits input; Vref input
function out = fcn(input_code, number_of_bits, Vref)
out = -Vref/2 + Vref/(2^number_of_bits) * (bi2de(input_code.', 'left-msb'));
end

== matlab function MMADC/Sensing Channel 1/SAR/ZOH+comparator/MATLAB Function ==
  data: SAR_clk_cycle input; y output
function y = fcn(SAR_clk_cycle)
    if (SAR_clk_cycle)==0
        y = 2;
    elseif (SAR_clk_cycle)==1
        y=3;
    else
        y=1;
    end
end

== matlab function MMADC/Sensing Channel 6/SAR/SAR/SAR ==
  data: output_code_decimal output size=1; cycle_out output size=1; output_code output size=number_of_bits; input_code_decimal input; cycle_in input; comparator_in input; number_of_bits input; done output; ZOH_true input
function [output_code_decimal, cycle_out, output_code, done] = fcn(input_code_decimal, cycle_in, comparator_in, number_of_bits, ZOH_true)

    input_code = de2bi(input_code_decimal, 'left-msb');
    output_code = [zeros(number_of_bits-size(input_code.',1),1); input_code.'];
    cycle_out = cycle_in + 1;
    done = 0;

    if (cycle_in < 2)
        
        % Wait for ZOH to be determined
        
    elseif (cycle_in == 2)
        % Reset output code, start SA algorithm unless ZOH
        if (~ZOH_true)
            output_code = zeros(number_of_bits,1);
            output_code(1, 1) = 1;
        end
        
    elseif (cycle_in == number_of_bits+2)
        % Finish SA algorithm unless ZOH, set done & reset output_cycle
        done = 1;
        if (~ZOH_true)
            output_code(number_of_bits,1) = comparator_in;
        end
        cycle_out = 0;
    else
        % Continue SA algorithm unless ZOH
        if (~ZOH_true)
            if (comparator_in == 0)
                output_code(cycle_in-2,1) = 0;
            end

            output_code(cycle_in-1,1) = 1;
        end
        
    end
    
    output_code_decimal_temp = bi2de(output_code.', 'left-msb');
    output_code_decimal = output_code_decimal_temp(1,1);
end

== matlab function MMADC/Sensing Channel 6/SAR/ZOH+comparator/MATLAB Function ==
  data: SAR_clk_cycle input; y output
function y = fcn(SAR_clk_cycle)
    if (SAR_clk_cycle)==0
        y = 2;
    elseif (SAR_clk_cycle)==1
        y=3;
    else
        y=1;
    end
end

== matlab function MMADC/Sensing Channel 7/SAR/DAC/DAC ==
  data: input_code input size=number_of_bits; out output double size=1; number_of_bits input; Vref input
function out = fcn(input_code, number_of_bits, Vref)
out = -Vref/2 + Vref/(2^number_of_bits) * (bi2de(input_code.', 'left-msb'));
end
